simulink model "patilass1"  (R2019a)
settings: Solver=FixedStepDiscrete  StartTime=0  StopTime=10  FixedStep=1  RelTol=1e-3
libraries: simulink x1
settings Model: Creator=Admin  LastModifiedBy=Admin

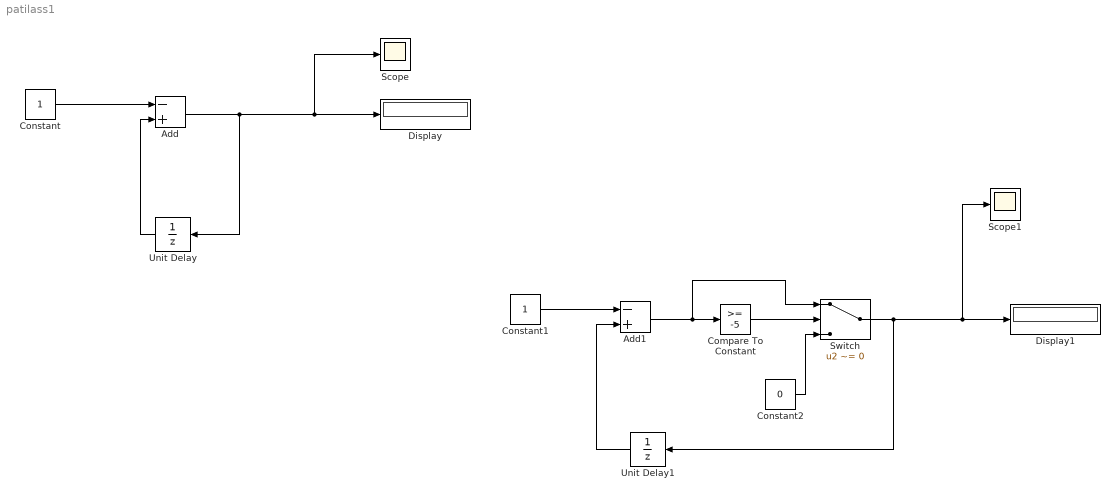
== system patilass1 ==
  Add : Sum  Inputs=-+
  Add1 : Sum  Inputs=-+
  Compare To Constant : simulink/Logic and Bit Operations/Compare To Constant  relop=>=  const=-5  OutDataTypeStr=boolean
  Constant : Constant
  Constant1 : Constant
  Constant2 : Constant  Value=0
  Display : Display
  Display1 : Display
  Scope : Scope
  Scope1 : Scope
  Switch : Switch  Criteria=u2 ~= 0
  Unit Delay : UnitDelay  InitialCondition=1  SampleTime=-1  HasFrameUpgradeWarning=on
  Unit Delay1 : UnitDelay  InitialCondition=1  SampleTime=-1  HasFrameUpgradeWarning=on
  wires:
  Constant/1 -> Add/1
  Add/1 -> Unit Delay/1, Scope/1, Display/1
  Unit Delay/1 -> Add/2
  Constant1/1 -> Add1/1
  Add1/1 -> Switch/1, Compare To Constant/1
  Compare To Constant/1 -> Switch/2
  Unit Delay1/1 -> Add1/2
  Switch/1 -> Unit Delay1/1, Scope1/1, Display1/1
  Constant2/1 -> Switch/3
